simulink model "CounterUpDownInlineFun"  (R2024b)
settings: Solver=VariableStepAuto  StartTime=0.0  StopTime=10.0  RelTol=1e-3
libraries: simulink x4
settings Model: SnapshotBufferSize=20  SnapshotInterval=20  Creator=vk09330  LastModifiedBy=z004f2se
settings DebuggingCC: UnderspecifiedInitializationDetection=Classic  MergeDetectMultiDrivingBlocksExec=none
settings ModelReferenceCC: PropagateSignalLabelsOutOfModel=off

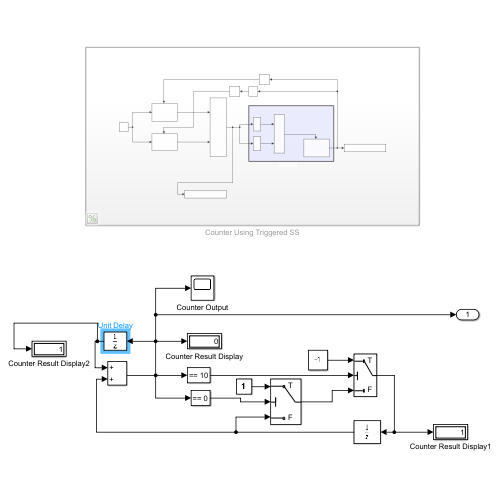
[thumbnail: Simulink's stored preview of the top-level diagram]
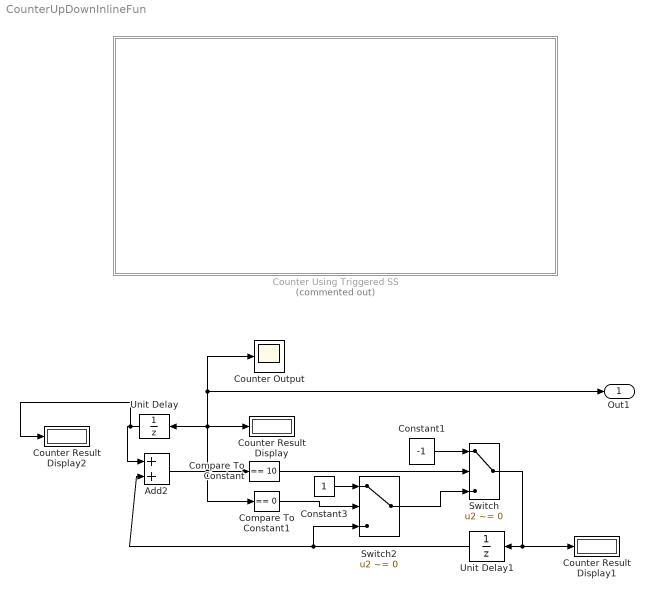
== system CounterUpDownInlineFun ==
  Add2 : Sum
  Compare To Constant : simulink/Logic and Bit Operations/Compare To Constant  relop===  const=10  OutDataTypeStr=boolean
  Compare To Constant1 : simulink/Logic and Bit Operations/Compare To Constant  relop===  const=0  OutDataTypeStr=boolean
  Constant1 : Constant  Value=-1
  Constant3 : Constant
  Counter Output : Scope
  Counter Result Display : Display
  Counter Result Display1 : Display
  Counter Result Display2 : Display
  Counter Using Triggered SS : Subsystem  Commented=on
  Switch : Switch  Criteria=u2 ~= 0  SaturateOnIntegerOverflow=off  InputSameDT=off
  Switch2 : Switch  Criteria=u2 ~= 0  SaturateOnIntegerOverflow=off  InputSameDT=off
  Unit Delay : UnitDelay  SampleTime=-1  HasFrameUpgradeWarning=on
  Unit Delay1 : UnitDelay  SampleTime=-1  HasFrameUpgradeWarning=on
  Out1 : Outport  VectorParamsAs1DForOutWhenUnconnected=off
  wires:
  Unit Delay1/1 -> Add2/2, Switch2/3
  Add2/1 -> Out1/1, Counter Output/1, Counter Result Display/1, Unit Delay/1, Compare To Constant/1, Compare To Constant1/1
  Unit Delay/1 -> Counter Result Display2/1, Add2/1
  Compare To Constant/1 -> Switch/2
  Constant1/1 -> Switch/1
  Constant3/1 -> Switch2/1
  Compare To Constant1/1 -> Switch2/2
  Switch2/1 -> Switch/3
  Switch/1 -> Counter Result Display1/1, Unit Delay1/1

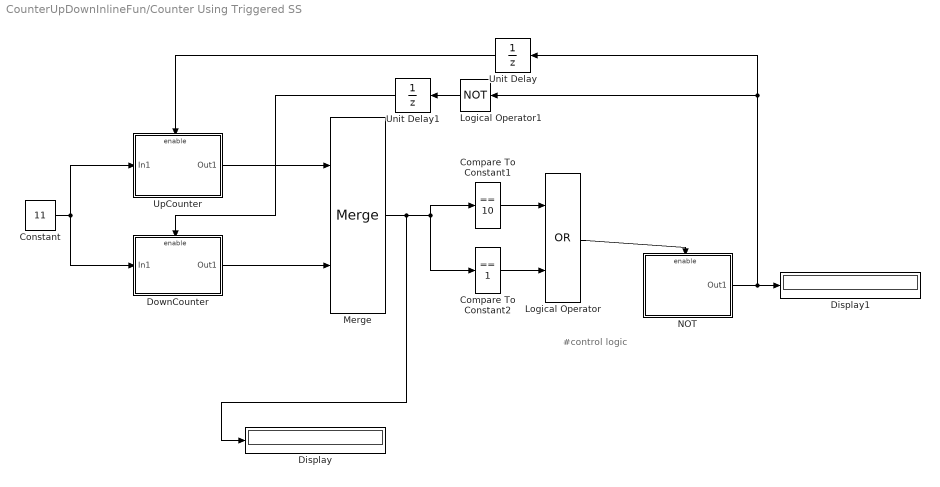
== system CounterUpDownInlineFun/Counter Using Triggered SS ==
  note: #control logic
  Compare To Constant1 : simulink/Logic and Bit Operations/Compare To Constant  relop===  const=10  OutDataTypeStr=boolean
  Compare To Constant2 : simulink/Logic and Bit Operations/Compare To Constant  relop===  const=1  OutDataTypeStr=boolean
  Constant : Constant  Value=11
  Display : Display
  Display1 : Display
  DownCounter : Subsystem  TreatAsAtomicUnit=on
      settings: RTWSystemCode=Inline
  Logical Operator : Logic  Operator=OR  AllPortsSameDT=off  OutDataTypeStr=boolean
  Logical Operator1 : Logic  Operator=NOT  AllPortsSameDT=off  OutDataTypeStr=boolean
  Merge : Merge
  NOT : Subsystem  TreatAsAtomicUnit=on
      settings: RTWSystemCode=Inline
  Unit Delay : UnitDelay  InitialCondition=1  SampleTime=-1  HasFrameUpgradeWarning=on
  Unit Delay1 : UnitDelay  SampleTime=-1  HasFrameUpgradeWarning=on
  UpCounter : Subsystem  TreatAsAtomicUnit=on
      settings: RTWSystemCode=Inline
  wires:
  Unit Delay/1 -> UpCounter/Enable
  Constant/1 -> UpCounter/1(In1), DownCounter/1(In1)
  Compare To Constant2/1 -> Logical Operator/2
  Unit Delay1/1 -> DownCounter/Enable
  Merge/1 -> Display/1, Compare To Constant2/1, Compare To Constant1/1
  UpCounter/1(Out1) -> Merge/1
  Logical Operator1/1 -> Unit Delay1/1
  Compare To Constant1/1 -> Logical Operator/1
  DownCounter/1(Out1) -> Merge/2
  NOT/1(Out1) -> Logical Operator1/1, Unit Delay/1, Display1/1
  Logical Operator/1 -> NOT/Enable

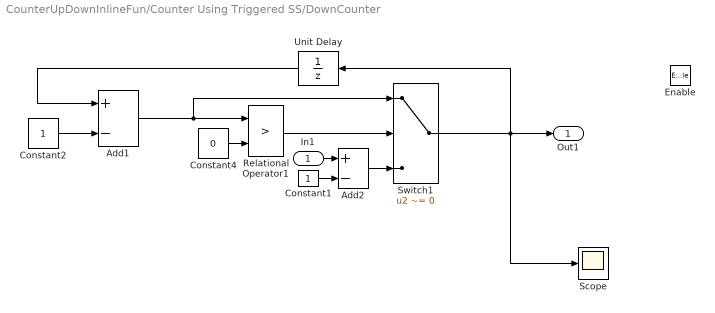
== system CounterUpDownInlineFun/Counter Using Triggered SS/DownCounter ==
  In1 : Inport
  Enable : EnablePort  StatesWhenEnabling=reset
  Add1 : Sum  Inputs=+-
  Add2 : Sum  Inputs=+-
  Constant1 : Constant
  Constant2 : Constant
  Constant4 : Constant  Value=0
  Relational Operator1 : RelationalOperator  Operator=>  OutDataTypeStr=boolean  RndMeth=Simplest  InputSameDT=off
  Scope : Scope
  Switch1 : Switch  Criteria=u2 ~= 0  SaturateOnIntegerOverflow=off  InputSameDT=off
  Unit Delay : UnitDelay  InitialCondition=9  SampleTime=-1  HasFrameUpgradeWarning=on
  Out1 : Outport  VectorParamsAs1DForOutWhenUnconnected=off
  wires:
  Constant2/1 -> Add1/2
  Constant4/1 -> Relational Operator1/2
  Relational Operator1/1 -> Switch1/2
  Add1/1 -> Relational Operator1/1, Switch1/1
  Unit Delay/1 -> Add1/1
  Switch1/1 -> Scope/1, Out1/1, Unit Delay/1
  In1/1 -> Add2/1
  Constant1/1 -> Add2/2
  Add2/1 -> Switch1/3

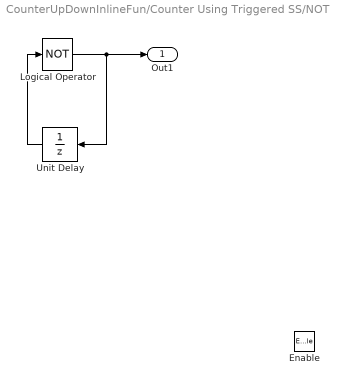
== system CounterUpDownInlineFun/Counter Using Triggered SS/NOT ==
  Enable : EnablePort
  Logical Operator : Logic  Operator=NOT  AllPortsSameDT=off  OutDataTypeStr=boolean
  Unit Delay : UnitDelay  SampleTime=-1  HasFrameUpgradeWarning=on
  Out1 : Outport  VectorParamsAs1DForOutWhenUnconnected=off
  wires:
  Unit Delay/1 -> Logical Operator/1
  Logical Operator/1 -> Unit Delay/1, Out1/1

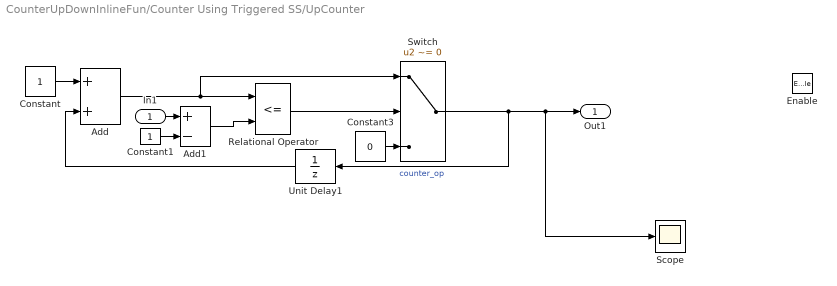
== system CounterUpDownInlineFun/Counter Using Triggered SS/UpCounter ==
  In1 : Inport
  Enable : EnablePort  StatesWhenEnabling=reset
  Add : Sum
  Add1 : Sum  Inputs=+-
  Constant : Constant
  Constant1 : Constant
  Constant3 : Constant  Value=0
  Relational Operator : RelationalOperator  Operator=<=  OutDataTypeStr=boolean  RndMeth=Simplest  InputSameDT=off
  Scope : Scope
  Switch : Switch  Criteria=u2 ~= 0  SaturateOnIntegerOverflow=off  InputSameDT=off
  Unit Delay1 : UnitDelay  SampleTime=-1  HasFrameUpgradeWarning=on
  Out1 : Outport  VectorParamsAs1DForOutWhenUnconnected=off
  wires:
  Constant/1 -> Add/1
  Add1/1 -> Relational Operator/2
  Relational Operator/1 -> Switch/2
  Switch/1 -> Unit Delay1/1, Scope/1, Out1/1  "counter_op"
  Constant3/1 -> Switch/3
  Add/1 -> Switch/1, Relational Operator/1
  Unit Delay1/1 -> Add/2
  In1/1 -> Add1/1
  Constant1/1 -> Add1/2
